simulink model "KR6_CLIK_Oval"  (R2018a)
settings: Solver=FixedStepAuto  StartTime=0.0  StopTime=100  FixedStep=0.01  RelTol=1e-3
libraries: vrlib x8, KR6_Lib x1, realtime_pacer_lib x1, simulink x1
settings Model: Creator=Pedro Ramalho  LastModifiedBy=Pedro Ramalho
settings DataIOCC: ReturnWorkspaceOutputs=on  ReturnWorkspaceOutputsName=qvectors

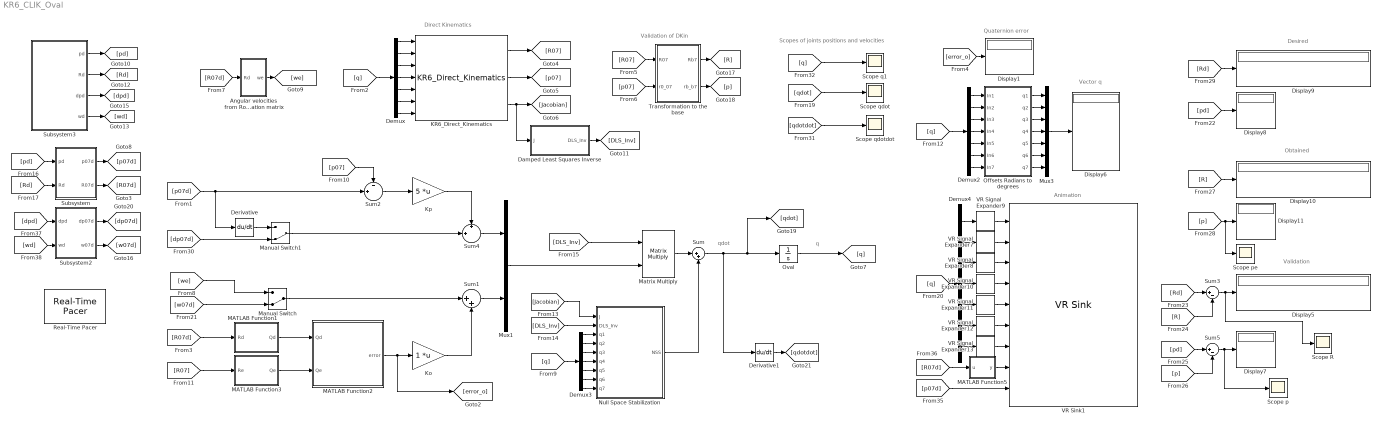
== system KR6_CLIK_Oval ==
  note: Direct Kinematics
  note: Validation of DKin
  note: qdot
  note: q
  note: Desired
  note: Obtained
  note: Validation
  note: Vector q
  note: Animation
  note: Scopes of joints positions and velocities
  note: Quaternion error
  Angular velocities from Rotation matrix : Subsystem
  Damped Least Squares Inverse : MATLAB Function  TreatAsAtomicUnit=on
  Demux{,2..4} (4 alike) : Demux  Outputs=7
  Derivative : Derivative
  Derivative1 : Derivative
  Display{1,5..11} (8 alike) : Display
  KR6_Direct_Kinematics : KR6_Lib/KR6_Direct_Kinematics
  Ko : Gain  Multiplication=Matrix(K*u)
  Kp : Gain  Gain=5  Multiplication=Matrix(K*u)
  MATLAB Function1 : MATLAB Function  TreatAsAtomicUnit=on
  MATLAB Function2 : MATLAB Function  TreatAsAtomicUnit=on
  MATLAB Function3 : MATLAB Function  TreatAsAtomicUnit=on
  MATLAB Function5 : MATLAB Function  TreatAsAtomicUnit=on
  Manual Switch : ManualSwitch  CurrentSetting=0
  Manual Switch1 : ManualSwitch  CurrentSetting=0
  Matrix Multiply : Product  Multiplication=Matrix(*)
  Mux1 : Mux  Inputs=2
  Mux3 : Mux  Inputs=7
  Null Space Stabilization : MATLAB Function  TreatAsAtomicUnit=on
  Offsets Radians to degrees : Subsystem
  Oval : Integrator  InitialCondition="[0.4246   -0.2313   -1.6935   -0.1482    0.7216    0.3543    4.0224]"  ZeroCross=off
  Real-Time Pacer : realtime_pacer_lib/Real-Time Pacer  simTimePerRealTime=1
  Scope R : Scope
  Scope p : Scope
  Scope pe : Scope
  Scope q1 : Scope
  Scope qdot : Scope
  Scope qdotdot : Scope
  Subsystem : Subsystem
  Subsystem2 : Subsystem
  Subsystem3 : Subsystem
  Sum : Sum  Inputs=|++
  Sum1 : Sum  Inputs=|++
  Sum2 : Sum  Inputs=-|+||
  Sum3 : Sum  Inputs=|+-
  Sum4 : Sum  Inputs=+|+||
  Sum5 : Sum  Inputs=|+-
  Transformation to the base : Subsystem
  VR Signal Expander{7..8,10..13} (6 alike) : vrlib/VR Signal Expander  outwidth=4  outidx=4
      settings: SourceProductName=Simulink 3D Animation  SourceProductBaseCode=VR
  VR Signal Expander9 : vrlib/VR Signal Expander  outwidth=3  outidx=3
      settings: SourceProductName=Simulink 3D Animation  SourceProductBaseCode=VR
  VR Sink1 : vrlib/VR Sink  InstantiateOnLoad=on  SampleTime=0.1  ViewEnable=on  RemoteChange=off  RemoteView=off  FieldsWritten=Jt1_DH_dv.translation.3.1.1.double#Jt2_DH_dv.rotation.4.1.1.double#Jt3_DH_dv.rotation.4.1.1.double#Jt4_DH_dv.rotation.4.1.1.double#Jt5_DH_dv.rotation.4.1.1.double#Jt6_DH_dv.rotation.4.1.1.double#Jt7_DH_dv.rotation.4.1.1.double#Desired.rotation.4.1.1.double#Desired.translation.3.1.1.double  WorldFileName=vrrobotKR6v2.wrl  WorldDescription=D-H Reference Frames for Virtual Reality Robot  AutoView=off  VideoDimensions=[]  AllowVariableSize=off
      settings: SourceProductBaseCode=VR
  wires:
  KR6_Direct_Kinematics/1 -> [R07]
  KR6_Direct_Kinematics/2 -> [p07]
  KR6_Direct_Kinematics/3 -> [Jacobian], Damped Least Squares Inverse/1(J)
  Demux/1 -> KR6_Direct_Kinematics/1
  Demux/2 -> KR6_Direct_Kinematics/2
  Demux/3 -> KR6_Direct_Kinematics/3
  Demux/4 -> KR6_Direct_Kinematics/4
  Demux/5 -> KR6_Direct_Kinematics/5
  Demux/6 -> KR6_Direct_Kinematics/6
  Demux/7 -> KR6_Direct_Kinematics/7
  [q] -> Demux/1
  [p07d] -> Sum2/2, Derivative/1
  Transformation to the base/2(rb_b7) -> [p]
  [R07] -> Transformation to the base/1(R07)
  [p07] -> Transformation to the base/2(r0_07)
  [R07d] -> MATLAB Function1/1(Rd)
  MATLAB Function1/1(Qd) -> MATLAB Function2/1(Qd)
  MATLAB Function2/1(error) -> [error_o], Ko/1
  Ko/1 -> Sum1/2
  Derivative/1 -> Manual Switch1/1
  [R07d] -> Angular velocities from Rotation matrix/1(Rd)
  Angular velocities from Rotation matrix/1(we) -> [we]
  [we] -> Manual Switch/1
  Manual Switch1/1 -> Sum4/2
  Kp/1 -> Sum4/1
  Manual Switch/1 -> Sum1/1
  Sum4/1 -> Mux1/1
  Sum1/1 -> Mux1/2
  [p07] -> Sum2/1
  [R07] -> MATLAB Function3/1(Re)
  MATLAB Function3/1(Qe) -> MATLAB Function2/2(Qe)
  Offsets Radians to degrees/5(q5) -> Mux3/5
  Demux2/4 -> Offsets Radians to degrees/4(In4)
  Offsets Radians to degrees/3(q3) -> Mux3/3
  [q] -> Demux2/1
  Demux2/3 -> Offsets Radians to degrees/3(In3)
  Offsets Radians to degrees/1(q1) -> Mux3/1
  Demux2/6 -> Offsets Radians to degrees/6(In6)
  Demux2/5 -> Offsets Radians to degrees/5(In5)
  Offsets Radians to degrees/7(q7) -> Mux3/7
  Offsets Radians to degrees/4(q4) -> Mux3/4
  Mux3/1 -> Display6/1
  Offsets Radians to degrees/2(q2) -> Mux3/2
  Demux2/2 -> Offsets Radians to degrees/2(In2)
  Demux2/1 -> Offsets Radians to degrees/1(In1)
  Offsets Radians to degrees/6(q6) -> Mux3/6
  Demux2/7 -> Offsets Radians to degrees/7(In7)
  Damped Least Squares Inverse/1(DLS_Inv) -> [DLS_Inv]
  Matrix Multiply/1 -> Sum/1
  Null Space Stabilization/1(NSS) -> Sum/2
  Mux1/1 -> Matrix Multiply/2
  [q] -> Demux3/1
  Demux3/5 -> Null Space Stabilization/7(q5)
  Demux3/7 -> Null Space Stabilization/9(q7)
  Demux3/2 -> Null Space Stabilization/4(q2)
  Demux3/1 -> Null Space Stabilization/3(q1)
  Demux3/3 -> Null Space Stabilization/5(q3)
  Demux3/4 -> Null Space Stabilization/6(q4)
  Demux3/6 -> Null Space Stabilization/8(q6)
  [Jacobian] -> Null Space Stabilization/1(J)
  [DLS_Inv] -> Null Space Stabilization/2(DLS_Inv)
  [DLS_Inv] -> Matrix Multiply/1
  [pd] -> Subsystem/1(pd)
  [Rd] -> Subsystem/2(Rd)
  Subsystem/1(p07d) -> [p07d]
  Subsystem/2(R07d) -> [R07d]
  Sum5/1 -> Scope p/1, Display7/1
  [Rd] -> Display9/1
  [R] -> Sum3/2
  Sum3/1 -> Scope R/1, Display5/1
  [p] -> Sum5/2
  [Rd] -> Sum3/1
  [pd] -> Sum5/1
  [p] -> Scope pe/1, Display11/1
  [pd] -> Display8/1
  [R] -> Display10/1
  Sum/1 -> Derivative1/1, [qdot], Oval/1
  Oval/1 -> [q]
  Sum2/1 -> Kp/1
  Transformation to the base/1(Rb7) -> [R]
  [qdot] -> Scope qdot/1
  Demux4/7 -> VR Signal Expander13/1
  Demux4/4 -> VR Signal Expander10/1
  Demux4/2 -> VR Signal Expander7/1
  Demux4/6 -> VR Signal Expander12/1
  Demux4/1 -> VR Signal Expander9/1
  [q] -> Demux4/1
  Demux4/5 -> VR Signal Expander11/1
  Demux4/3 -> VR Signal Expander8/1
  [error_o] -> Display1/1
  [p07d] -> VR Sink1/9
  [R07d] -> MATLAB Function5/1(u)
  MATLAB Function5/1(y) -> VR Sink1/8
  [dpd] -> Subsystem2/1(dpd)
  [wd] -> Subsystem2/2(wd)
  Subsystem2/1(dp07d) -> [dp07d]
  Subsystem2/2(w07d) -> [w07d]
  Derivative1/1 -> [qdotdot]
  [qdotdot] -> Scope qdotdot/1
  [q] -> Scope q1/1
  VR Signal Expander9/1 -> VR Sink1/1
  VR Signal Expander7/1 -> VR Sink1/2
  VR Signal Expander8/1 -> VR Sink1/3
  VR Signal Expander10/1 -> VR Sink1/4
  VR Signal Expander11/1 -> VR Sink1/5
  VR Signal Expander12/1 -> VR Sink1/6
  VR Signal Expander13/1 -> VR Sink1/7
  Subsystem3/1(pd) -> [pd]
  Subsystem3/2(Rd) -> [Rd]
  Subsystem3/3(dpd) -> [dpd]
  Subsystem3/4(wd) -> [wd]
  [dp07d] -> Manual Switch1/2
  [w07d] -> Manual Switch/2

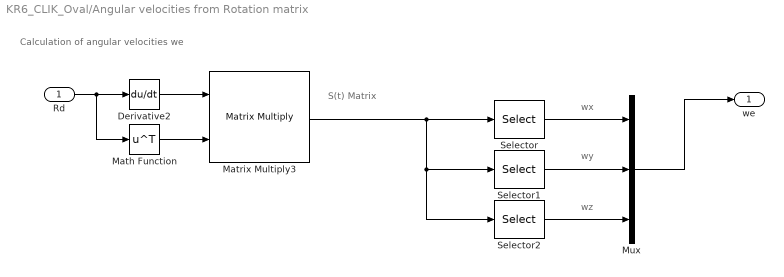
== system KR6_CLIK_Oval/Angular velocities from Rotation matrix ==
  note: S(t) Matrix
  note: wx
  note: Calculation of angular velocities we
  note: wz
  note: wy
  Rd : Inport
  Derivative2 : Derivative
  Math Function : Math  Operator=transpose  SaturateOnIntegerOverflow=on
  Matrix Multiply3 : Product  Multiplication=Matrix(*)
  Mux : Mux  Inputs=3
  Selector : Selector  NumberOfDimensions=2  InputPortWidth=3  IndexOptions=Index vector (dialog),Index vector (dialog)  Indices=[3],[2]  OutputSizes=1,1
  Selector1 : Selector  NumberOfDimensions=2  InputPortWidth=3  IndexOptions=Index vector (dialog),Index vector (dialog)  Indices=[1],[3]  OutputSizes=1,1
  Selector2 : Selector  NumberOfDimensions=2  InputPortWidth=3  IndexOptions=Index vector (dialog),Index vector (dialog)  Indices=[2],[1]  OutputSizes=1,1
  we : Outport
  wires:
  Mux/1 -> we/1
  Matrix Multiply3/1 -> Selector2/1, Selector1/1, Selector/1
  Rd/1 -> Math Function/1, Derivative2/1
  Derivative2/1 -> Matrix Multiply3/1
  Math Function/1 -> Matrix Multiply3/2
  Selector1/1 -> Mux/2
  Selector/1 -> Mux/1
  Selector2/1 -> Mux/3

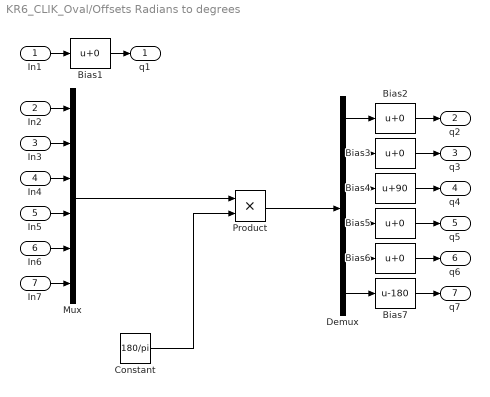
== system KR6_CLIK_Oval/Offsets Radians to degrees ==
  In1 : Inport
  In2 : Inport  Port=2
  In3 : Inport  Port=3
  In4 : Inport  Port=4
  In5 : Inport  Port=5
  In6 : Inport  Port=6
  In7 : Inport  Port=7
  Bias{1..3,5..6} (5 alike) : Bias
  Bias4 : Bias  Bias=90
  Bias7 : Bias  Bias=-180
  Constant : Constant  Value=180/pi
  Demux : Demux  Outputs=6
  Mux : Mux  Inputs=6
  Product : Product
  q1 : Outport
  q2 : Outport  Port=2
  q3 : Outport  Port=3
  q4 : Outport  Port=4
  q5 : Outport  Port=5
  q6 : Outport  Port=6
  q7 : Outport  Port=7
  wires:
  In1/1 -> Bias1/1
  Bias1/1 -> q1/1
  Mux/1 -> Product/1
  Constant/1 -> Product/2
  Product/1 -> Demux/1
  In2/1 -> Mux/1
  In3/1 -> Mux/2
  In4/1 -> Mux/3
  In5/1 -> Mux/4
  In6/1 -> Mux/5
  In7/1 -> Mux/6
  Demux/1 -> Bias2/1
  Demux/2 -> Bias3/1
  Demux/3 -> Bias4/1
  Demux/4 -> Bias5/1
  Demux/5 -> Bias6/1
  Demux/6 -> Bias7/1
  Bias2/1 -> q2/1
  Bias3/1 -> q3/1
  Bias4/1 -> q4/1
  Bias5/1 -> q5/1
  Bias6/1 -> q6/1
  Bias7/1 -> q7/1

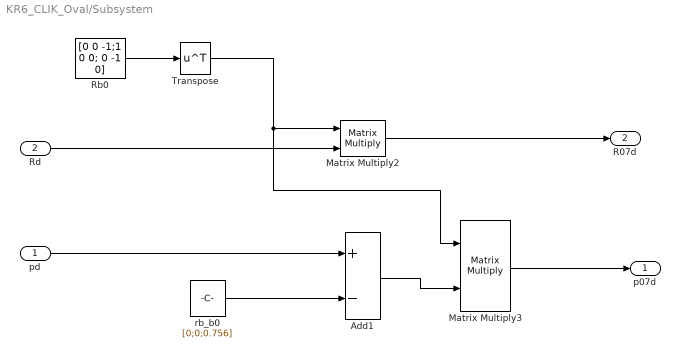
== system KR6_CLIK_Oval/Subsystem ==
  pd : Inport
  Rd : Inport  Port=2
  Add1 : Sum  Inputs=+-
  Matrix Multiply2 : Product  Multiplication=Matrix(*)
  Matrix Multiply3 : Product  Multiplication=Matrix(*)
  Rb0 : Constant  Value=[0 0 -1;1 0 0; 0 -1 0]
  Transpose : Math  Operator=transpose  SaturateOnIntegerOverflow=on
  rb_b0 : Constant  Value=[0;0;0.756]
  p07d : Outport
  R07d : Outport  Port=2
  wires:
  Add1/1 -> Matrix Multiply3/2
  Matrix Multiply3/1 -> p07d/1
  Rb0/1 -> Transpose/1
  Transpose/1 -> Matrix Multiply3/1, Matrix Multiply2/1
  Rd/1 -> Matrix Multiply2/2
  rb_b0/1 -> Add1/2
  pd/1 -> Add1/1
  Matrix Multiply2/1 -> R07d/1

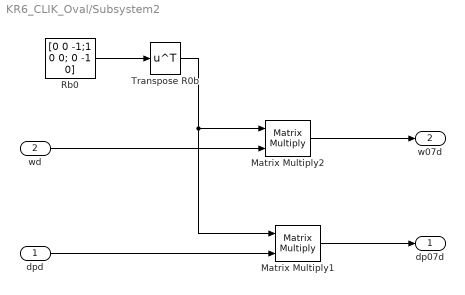
== system KR6_CLIK_Oval/Subsystem2 ==
  dpd : Inport
  wd : Inport  Port=2
  Matrix Multiply1 : Product  Multiplication=Matrix(*)
  Matrix Multiply2 : Product  Multiplication=Matrix(*)
  Rb0 : Constant  Value=[0 0 -1;1 0 0; 0 -1 0]
  Transpose R0b : Math  Operator=transpose  SaturateOnIntegerOverflow=on
  dp07d : Outport
  w07d : Outport  Port=2
  wires:
  Matrix Multiply1/1 -> dp07d/1
  Rb0/1 -> Transpose R0b/1
  Transpose R0b/1 -> Matrix Multiply2/1, Matrix Multiply1/1
  wd/1 -> Matrix Multiply2/2
  dpd/1 -> Matrix Multiply1/2
  Matrix Multiply2/1 -> w07d/1

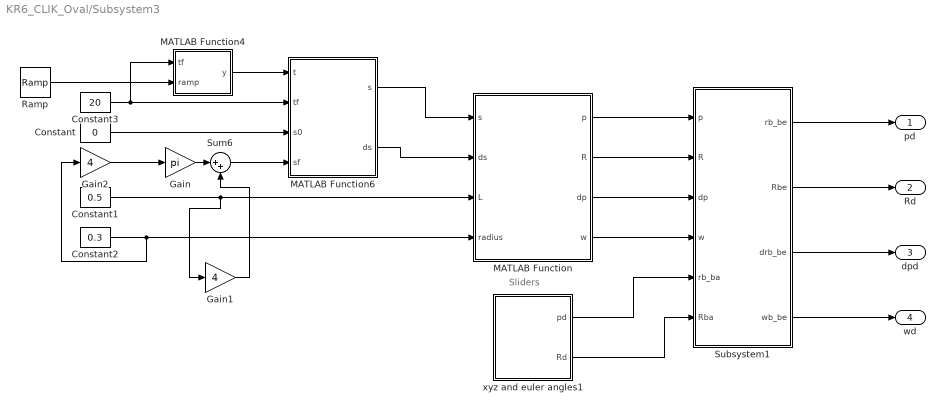
== system KR6_CLIK_Oval/Subsystem3 ==
  note: Sliders
  Constant : Constant  Value=0
  Constant1 : Constant  Value=0.5
  Constant2 : Constant  Value=0.3
  Constant3 : Constant  Value=20
  Gain : Gain  Gain=pi
  Gain1 : Gain  Gain=4
  Gain2 : Gain  Gain=4
  MATLAB Function : MATLAB Function  TreatAsAtomicUnit=on
  MATLAB Function4 : MATLAB Function  TreatAsAtomicUnit=on
  MATLAB Function6 : MATLAB Function  TreatAsAtomicUnit=on
  Ramp : simulink/Sources/Ramp  slope=1  start=0  InitialOutput=0
  Subsystem1 : Subsystem
  Sum6 : Sum  Inputs=|++
  xyz and euler angles1 : Subsystem  mask{px=-0.5, py=0.5, pz=1.2, phi=0, theta=0, psi=90}
      mask prompts: px "x"; py "y"; pz "z"
      mask DialogControl ParameterGroupVar_copy Prompt: Euler angles
  pd : Outport
  Rd : Outport  Port=2
  dpd : Outport  Port=3
  wd : Outport  Port=4
  wires:
  Constant/1 -> MATLAB Function6/3(s0)
  Constant2/1 -> Gain2/1, MATLAB Function/4(radius)
  Ramp/1 -> MATLAB Function4/2(ramp)
  MATLAB Function/1(p) -> Subsystem1/1(p)
  Constant1/1 -> Gain1/1, MATLAB Function/3(L)
  Constant3/1 -> MATLAB Function6/2(tf), MATLAB Function4/1(tf)
  Gain/1 -> Sum6/1
  Gain2/1 -> Gain/1
  MATLAB Function/4(w) -> Subsystem1/4(w)
  xyz and euler angles1/1(pd) -> Subsystem1/5(rb_ba)
  xyz and euler angles1/2(Rd) -> Subsystem1/6(Rba)
  MATLAB Function/2(R) -> Subsystem1/2(R)
  MATLAB Function4/1(y) -> MATLAB Function6/1(t)
  MATLAB Function/3(dp) -> Subsystem1/3(dp)
  MATLAB Function6/2(ds) -> MATLAB Function/2(ds)
  MATLAB Function6/1(s) -> MATLAB Function/1(s)
  Gain1/1 -> Sum6/2
  Sum6/1 -> MATLAB Function6/4(sf)
  Subsystem1/2("Rbe ") -> Rd/1
  Subsystem1/3("drb_be ") -> dpd/1
  Subsystem1/1("rb_be ") -> pd/1
  Subsystem1/4(wb_be) -> wd/1

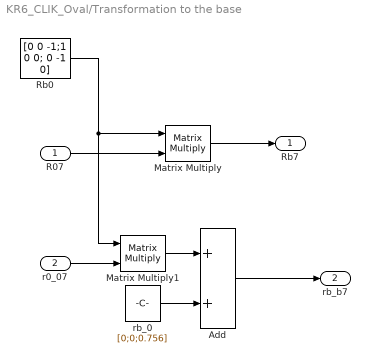
== system KR6_CLIK_Oval/Transformation to the base ==
  R07 : Inport
  r0_07 : Inport  Port=2
  Add : Sum
  Matrix Multiply : Product  Multiplication=Matrix(*)
  Matrix Multiply1 : Product  Multiplication=Matrix(*)
  Rb0 : Constant  Value=[0 0 -1;1 0 0; 0 -1 0]
  rb_0 : Constant  Value=[0;0;0.756]
  Rb7 : Outport
  rb_b7 : Outport  Port=2
  wires:
  Matrix Multiply1/1 -> Add/1
  R07/1 -> Matrix Multiply/2
  rb_0/1 -> Add/2
  Rb0/1 -> Matrix Multiply1/1, Matrix Multiply/1
  Matrix Multiply/1 -> Rb7/1
  r0_07/1 -> Matrix Multiply1/2
  Add/1 -> rb_b7/1

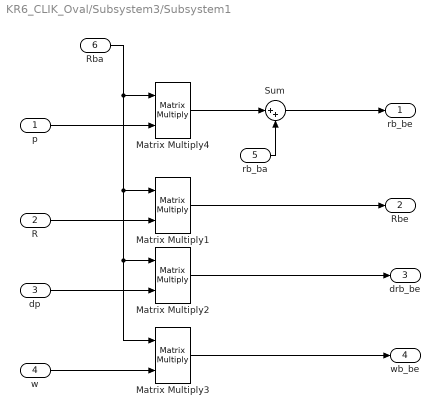
== system KR6_CLIK_Oval/Subsystem3/Subsystem1 ==
  p : Inport
  R : Inport  Port=2
  dp : Inport  Port=3
  w : Inport  Port=4
  rb_ba : Inport  Port=5
  Rba : Inport  Port=6
  Matrix Multiply{1..4} (4 alike) : Product  Multiplication=Matrix(*)
  Sum : Sum  Inputs=|++
  "rb_be " : Outport
  "Rbe " : Outport  Port=2
  "drb_be " : Outport  Port=3
  wb_be : Outport  Port=4
  wires:
  rb_ba/1 -> Sum/2
  w/1 -> Matrix Multiply3/2
  dp/1 -> Matrix Multiply2/2
  Matrix Multiply2/1 -> "drb_be "/1
  Matrix Multiply3/1 -> wb_be/1
  Sum/1 -> "rb_be "/1
  R/1 -> Matrix Multiply1/2
  Matrix Multiply1/1 -> "Rbe "/1
  p/1 -> Matrix Multiply4/2
  Rba/1 -> Matrix Multiply4/1, Matrix Multiply1/1, Matrix Multiply3/1, Matrix Multiply2/1
  Matrix Multiply4/1 -> Sum/1

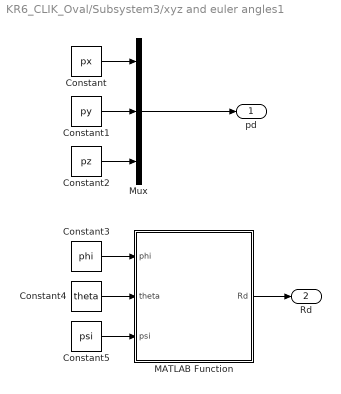
== system KR6_CLIK_Oval/Subsystem3/xyz and euler angles1 ==
  Constant : Constant  Value=px
  Constant1 : Constant  Value=py
  Constant2 : Constant  Value=pz
  Constant3 : Constant  Value=phi
  Constant4 : Constant  Value=theta
  Constant5 : Constant  Value=psi
  MATLAB Function : MATLAB Function  TreatAsAtomicUnit=on
  Mux : Mux  Inputs=3
  pd : Outport
  Rd : Outport  Port=2
  wires:
  Constant/1 -> Mux/1
  Constant1/1 -> Mux/2
  Constant2/1 -> Mux/3
  Mux/1 -> pd/1
  Constant3/1 -> MATLAB Function/1(phi)
  Constant4/1 -> MATLAB Function/2(theta)
  Constant5/1 -> MATLAB Function/3(psi)
  MATLAB Function/1(Rd) -> Rd/1

== matlab function KR6_CLIK_Oval/Subsystem3/MATLAB Function ==
  data: s input; ds input; p output; L input; radius input; R output; dp output; w output
function [p,R,dp,w] = trajectory(s,ds,L,radius)

p = [0;0;0];
R = rotx(180);
dp = [0;0;0];
w = [0;0;0];

if (0 <= s) && (s <= L)
    p = [s;0;0];
    R = rotx(180);
    dp = [ds;0;0];
    w = [0;0;0];
elseif (L < s) && (s <= L+pi*radius)
    theta = (s-L)/radius;
    p = [L+radius*sin(theta);-radius+radius*cos(theta);0];
    Rz = [cos(theta),-sin(theta),0;
          sin(theta), cos(theta),0;
          0,0,1];
    R = rotx(180)*Rz;
    dp = [ds*cos(theta);-ds*sin(theta)*1.21;0];
    dRz = (ds/radius)*[-sin(theta),-cos(theta),0;
                        cos(theta),-sin(theta),0;
                        0,0,1];
    Sw = rotx(180)*dRz*Rz'*rotx(180)';
    w = [Sw(3,2);Sw(1,3);Sw(2,1)];

elseif (L+pi*radius < s) && (s <= 2*L+pi*radius)
    p = [L+(L+pi*radius)-s;-2*radius;0];
    R = rotx(180)*rotz(180);
    dp = [-ds;0;0];
    w = [0;0;0];
    
elseif (2*L+pi*radius < s) && (s <= 2*L+2*pi*radius)
    theta = pi+(s-(2*L+pi*radius))/radius;
    p = [radius*sin(theta);-radius+radius*cos(theta);0];
    Rz = [cos(theta),-sin(theta),0;
          sin(theta), cos(theta),0;
          0,0,1];
    R = rotx(180)*Rz;
    dp = [ds*cos(theta);-ds*sin(theta)*1.21;0];
    dRz = (ds/radius)*[-sin(theta),-cos(theta),0;
                        cos(theta),-sin(theta),0;
                        0,0,1];
    Sw = rotx(180)*dRz*Rz'*rotx(180)';
    w = [Sw(3,2);Sw(1,3);Sw(2,1)]; 
    
elseif (2*L+2*pi*radius < s) && (s <= 3*L+2*pi*radius) 
    p = [s-(2*L+2*pi*radius);0;0];
    R = rotx(180);
    dp = [ds;0;0];
    w = [0;0;0];

elseif (3*L+2*pi*radius < s) && (s <= 3*L+3*pi*radius)
    theta = (s-(3*L+2*pi*radius))/radius;
    p = [L+radius*sin(theta);-radius+radius*cos(theta);0];
    Rz = [cos(theta),-sin(theta),0;
          sin(theta), cos(theta),0;
          0,0,1];
    R = rotx(180)*Rz;
    dp = [ds*cos(theta);-ds*sin(theta)*1.21;0];
    dRz = (ds/radius)*[-sin(theta),-cos(theta),0;
                        cos(theta),-sin(theta),0;
                        0,0,1];
    Sw = rotx(180)*dRz*Rz'*rotx(180)';
    w = [Sw(3,2);Sw(1,3);Sw(2,1)];
    
elseif (3*L+3*pi*radius < s) && (s <= 4*L+3*pi*radius)
    p = [L+(3*L+3*pi*radius)-s;-2*radius;0];
    R = rotx(180)*rotz(180);
    dp = [-ds;0;0];
    w = [0;0;0];
    
elseif (4*L+3*pi*radius < s) && (s <= 4*L+4*pi*radius)
    theta = pi+(s-(4*L+3*pi*radius))/radius;
    p = [radius*sin(theta);-radius+radius*cos(theta);0];
    Rz = [cos(theta),-sin(theta),0;
          sin(theta), cos(theta),0;
          0,0,1];
    R = rotx(180)*Rz;
    dp = [ds*cos(theta);-ds*sin(theta)*1.21;0];
    dRz = (ds/radius)*[-sin(theta),-cos(theta),0;
                        cos(theta),-sin(theta),0;
                        0,0,1];
    Sw = rotx(180)*dRz*Rz'*rotx(180)';
    w = [Sw(3,2);Sw(1,3);Sw(2,1)]; 
    
end

== matlab function KR6_CLIK_Oval/MATLAB Function3 ==
  data: Re input; Qe output
function Qe = fcn(Re)


Qe=rotm2quat(Re);

== matlab function KR6_CLIK_Oval/Subsystem3/MATLAB Function4 ==
  data: tf input; ramp input; y output
function y = time(tf,ramp)

y = ramp;
%c = tf-2.5;
if ramp > tf
    y = ramp - (tf)*floor(ramp/(tf));
end

== matlab function KR6_CLIK_Oval/Damped Least Squares Inverse ==
  data: J input size=[6 7]; DLS_Inv output
function DLS_Inv = fcn(J)
Jt = transpose(J);
k = 0.1;
%k = 0.1;
DLS_Inv = Jt/(J*Jt + k^2*eye(6));

== matlab function KR6_CLIK_Oval/MATLAB Function1 ==
  data: Rd input; Qd output
function Qd = fcn(Rd)


Qd=rotm2quat(Rd);

== matlab function KR6_CLIK_Oval/MATLAB Function2 ==
  data: Qd input; error output; Qe input
function error = ErrorComput(Qd, Qe)


error=Qe(1)*Qd(2:4)-Qd(1)*Qe(2:4)-cross(Qd(2:4),Qe(2:4));

== matlab function KR6_CLIK_Oval/Null Space Stabilization ==
  data: J input; DLS_Inv input; q1 input; NSS output; q2 input; q3 input; q4 input; q5 input; q6 input; q7 input
function NSS = fcn(J,DLS_Inv,q1,q2,q3,q4,q5,q6,q7)

qdot0 = [-(8100*q1)/(7*pi^2)/50; %50
     -(81*q2)/(2023*pi^2);
   -(2*q3 + pi)/(56*pi^2);
     -(81*q4)/(2023*pi^2);
    -(324*q5)/(9583*pi^2);
       -(9*q6)/(112*pi^2);
 -(2*q7 - 2*pi)/(56*pi^2)];

k0 = 0.01;
%k0 = 0.01;
NSS = (eye(7)- DLS_Inv * J)*qdot0*k0;

== matlab function KR6_CLIK_Oval/MATLAB Function5 ==
  data: u input; y output
function y = fcn(u)
y=rotm2axang(u);

== matlab function KR6_CLIK_Oval/Subsystem3/MATLAB Function6 ==
  data: t input; s output; tf input; s0 input; sf input; ds output
function [s,ds] = time_law(t,tf,s0,sf)

s = s0 + 3*(sf-s0)*(t/tf)^2 - 2*(sf-s0)*(t/tf)^3;
ds = (6/tf^2)*(sf-s0)*t - (6/tf^3)*(sf-s0)*t^2;

== matlab function KR6_CLIK_Oval/Subsystem3/xyz and euler angles1/MATLAB Function ==
  data: phi input; Rd output; theta input; psi input
function Rd = fcn(phi,theta,psi)

eul = pi/180*[phi theta psi];
Rd = eul2rotm(eul);

end
